simulink model "GCI_Ctrl_PLL_C2000"  (R2024a)
settings: Solver=FixedStepDiscrete  StartTime=0.0  StopTime=8  FixedStep=Sim.ContSampleTime  RelTol=1e-3  EnableMultiTasking=on
values from neighbouring files (symbols this model uses):
  ADPTV = 1.3912    [ModelDD.sldd]
  Ctrl = 0    [ModelDD.sldd]
  EnableMonitors = 0    [ModelDD.sldd]
  FrcPwr = 1    [ModelDD.sldd]
  IdSp = 0.0    [ModelDD.sldd]
  IqSp = 0.0    [ModelDD.sldd]
  ModReq = 1    [ModelDD.sldd]
  PorISel = 0    [ModelDD.sldd]
  PSp = 0.0    [ModelDD.sldd]
  QSp = 0.0    [ModelDD.sldd]
  Sim : value not decoded    [ModelDD.sldd]
  Test = 0    [ModelDD.sldd]
  Var = 650.0    [ModelDD.sldd]
undefined symbols (not defined in the file or in its folder): DiscIntNeverNeededParam, Down, GPTRIP1SEL, GPTRIP2SEL, magnitude, P, TZ1, TZ2, Up
libraries: simulink x38, c2837xDlib x22, c2802xlib x15, slpidlib x9, spsMeanLib x9, spsCurrentMeasurementLib x7, spsThreePhaseVIMeasurementLib x5, spsVoltageMeasurementLib x5, spsTHDLib x4, spsSeriesRLCBranchLib x4, svdutilitieslib x3, c280xlib x3
(part 2 of 11)

== system GCI_Ctrl_PLL_C2000/PowerSystem/Plant ==
  DutyIn : Inport
  Current Measurement : spsCurrentMeasurementLib/Current Measurement  PhasorSimulation=off  OutputType=Complex  PSBequivalent=0
  Current Measurement1 : spsCurrentMeasurementLib/Current Measurement  PhasorSimulation=off  OutputType=Complex  PSBequivalent=0
  Current Measurement2 : spsCurrentMeasurementLib/Current Measurement  PhasorSimulation=off  OutputType=Complex  PSBequivalent=0
  DC Voltage Source : spsDCVoltageSourceLib/DC Voltage Source  Amplitude=double(Var.HVDC.V)  Measurements=Voltage
  Data Type Conversion : DataTypeConversion  SaturateOnIntegerOverflow=off  RndMeth=Floor
  Data Type Conversion1 : DataTypeConversion  SaturateOnIntegerOverflow=off  RndMeth=Floor
  Ground : Ground
  Ground1 : spsGroundLib/Ground  LConnTagsString=a
  Measurment : Subsystem
  PWMGen1 : Subsystem  Commented=on  VariantControl=Var.Sim.SimOrHw == 1
  PWMGen2 : Subsystem  VariantControl=Var.Sim.SimOrHw == 1
  Series RLC Branch : spsSeriesRLCBranchLib/Series RLC Branch  LConnTagsString=__new0  RConnTagsString=__new0  BranchType=RC  Resistance=double(Var.HVDC.Cesr)  Inductance=1e-3  SetiL0=off  InitialCurrent=0  Capacitance=double(Var.HVDC.C)  Setx0=off  InitialVoltage=0  Measurements=Branch voltage and current
  Series RLC Branch1 : spsSeriesRLCBranchLib/Series RLC Branch  LConnTagsString=__new0  RConnTagsString=__new0  BranchType=RL  Resistance=double(Var.HVDC.Lesr)  Inductance=double(Var.HVDC.L)  SetiL0=off  InitialCurrent=0  Capacitance=Var.HVDC.C  Setx0=off  InitialVoltage=0  Measurements=Branch voltage and current
  Three-Phase Programmable Voltage Source1 : spsThreePhaseProgrammableVoltageSourceLib/Three-Phase Programmable Voltage Source  PositiveSequence="[double(Var.Grid.VphRms)*sqrt(3)  0 double(Var.Grid.Frq)]"  VariationEntity=Amplitude  VariationType=Table of time-amplitude pairs  VariationTypeAlt=Step  VariationStep=-20  VariationRate=10  VariationMagnitude=0.3  VariationFrequency=2  VariationTiming=[1 2]  VariationPhaseA=on  Amplitudes=[1 0.2 1]  TimeValues=[0 0.1 100]  HarmonicGeneration=on  HarmonicA=[3 0.05 -25 0]  HarmonicB=[5 0.05 35 0]  Timing="[0  110]"  BusType=swing  Pref=0  Qref=0  Qmin=-inf  Qmax=inf
  Three-Phase Series RLC Branch : spsThreePhaseSeriesRLCBranchLib/Three-Phase Series RLC Branch  LConnTagsString=A|B|C  RConnTagsString=A|B|C  BranchType=RL  Resistance=double(Var.Inductor.R)  Inductance=double(Var.Inductor.L)  Capacitance=1e-6  Measurements=Branch voltages and currents
  Three-Phase V-I Measurement1 : spsThreePhaseVIMeasurementLib/Three-Phase V-I Measurement  VoltageMeasurement=phase-to-ground  SetLabelV=on  LabelV=Vgrid_Ls  Vpu=off  VpuLL=off  CurrentMeasurement=no  SetLabelI=off  LabelI=Igrid_Ls  Ipu=off  Pbase=100e6  Vbase=500e3  OutputType=Complex  PhasorSimulation=off  PSBequivalent=0
  Three-Phase V-I Measurement4 : spsThreePhaseVIMeasurementLib/Three-Phase V-I Measurement  VoltageMeasurement=phase-to-ground  SetLabelV=on  LabelV=Vinv  Vpu=off  VpuLL=off  CurrentMeasurement=yes  SetLabelI=on  LabelI=Iinv  Ipu=off  Pbase=100e6  Vbase=500e3  OutputType=Complex  PhasorSimulation=off  PSBequivalent=0
  Two-Level Converter : spsTwoLevelConverterLib/Two-Level Converter  ModelType=Switching devices  Ron=1e-3  Rs=1e6  Cs=inf  Vforward=[0,0]  Ron_Diode=1e-3  Rs_Diode=1e6  Cs_Diode=inf  Vf_Diode=1e-3  Rs_CurrentSource=inf  Ron_ACsource=1e-3
      settings: LibrarySourceBlock=sps_lib/Power Electronics/Two-Level Converter
  Voltage Measurement : spsVoltageMeasurementLib/Voltage Measurement  PhasorSimulation=off  OutputType=Complex  PSBequivalent=0
  Voltage Measurement1 : spsVoltageMeasurementLib/Voltage Measurement  PhasorSimulation=off  OutputType=Complex  PSBequivalent=0
  powergui1 : spspowerguiLib/powergui  Priority=1  SimulationMode=Discrete  SampleTime=Sim.ContSampleTime  frequency=60  Iterations=50  frequencyindice=0  Pbase=100e6  ErrMax=1e-4  UnitsV=kV  UnitsW=MW  buscounter=0  FunctionMessages=off  echomessages=off  EnableUseOfTLC=off  CurrentSourceSwitches=off  DisableSnubberDevices=off  DisableRonSwitches=off  DisableVfSwitches=off  DisplayEquations=off  AutomaticDiscreteSolvers=off  SolverType=Tustin/Backward Euler (TBE)  Interpol=off  ExternalGateDelay=off  methode=off  Ts=100  x0status=blocks  SPID=off  SwTol=0  HookPort=off  NonlinearTolerance=1e-4  nMaxIteration=100  ContinueOnMaxIteration=off  RestoreLinks=warning  ResistiveCurrentMeasurement=off  Frange=[0:2:500]  Ylog=off  Xlog=on  ShowGrid=off  save=off  variable=ZData  structure=ScopeData2  ZoomFFT=off  StartTime=4.2  cycles=50  DisplayStyle=3  fundamental=46.5  FreqAxis=on  MaxFrequency=inf  frequencyindicesteady=1  RmsSteady=1  display=off
  MCU : Outport  VectorParamsAs1DForOutWhenUnconnected=off
  wires:
  [Vbat] -> Measurment/7(Vbat)
  [IhvdcCap] -> Measurment/6(Ihvdc_capa)
  Voltage Measurement/1 -> [Vbat]
  Data Type Conversion/1 -> MCU/1
  Current Measurement1/1 -> [IhvdcCap]
  [Ibat] -> Measurment/8(Ibat)
  [Vinv] -> Measurment/4(Vinv_abc)  "Vinv_abc"
  Measurment/1(MCU) -> Data Type Conversion/1
  [Ihvdc] -> Measurment/3(I_HVDC)  "I_HVD"
  [Vhvdc] -> Measurment/2(V_HVDC)  "V_HVD"
  [Vgrid_Ls] -> Measurment/1(Vgrid_abc)  "Vgrid_abc"
  DutyIn/1 -> PWMGen2/1(Duty)
  Data Type Conversion1/1 -> Two-Level Converter/1
  Ground/1 -> Two-Level Converter/2
  Current Measurement/1 -> [Ihvdc]
  Voltage Measurement1/1 -> [Vhvdc]
  [Iinv] -> Measurment/5(Iinv_abc)  "Iinv_abc"
  Current Measurement2/1 -> [Ibat]
  PWMGen2/1(PWM) -> Data Type Conversion1/1
  connections:
  Three-Phase V-I Measurement4/RConn1 -- Three-Phase Series RLC Branch/LConn1
  Three-Phase V-I Measurement1/RConn1 -- Three-Phase Series RLC Branch/RConn1
  DC Voltage Source/LConn1 -- Voltage Measurement1/LConn2 -- Voltage Measurement/LConn2 -- Series RLC Branch/RConn1 -- Two-Level Converter/RConn2
  Current Measurement/RConn1 -- Two-Level Converter/RConn1
  Three-Phase V-I Measurement4/LConn3 -- Two-Level Converter/LConn3
  Three-Phase V-I Measurement4/RConn2 -- Three-Phase Series RLC Branch/LConn2
  Three-Phase V-I Measurement1/RConn3 -- Three-Phase Series RLC Branch/RConn3
  Three-Phase V-I Measurement1/RConn2 -- Three-Phase Series RLC Branch/RConn2
  Current Measurement2/LConn1 -- Series RLC Branch1/RConn1
  DC Voltage Source/RConn1 -- Series RLC Branch1/LConn1 -- Voltage Measurement/LConn1
  Current Measurement/LConn1 -- Voltage Measurement1/LConn1 -- Current Measurement2/RConn1 -- Current Measurement1/LConn1
  Three-Phase V-I Measurement4/LConn1 -- Two-Level Converter/LConn1
  Three-Phase V-I Measurement4/LConn2 -- Two-Level Converter/LConn2
  Current Measurement1/RConn1 -- Series RLC Branch/LConn1
  Three-Phase V-I Measurement4/RConn3 -- Three-Phase Series RLC Branch/LConn3
  Three-Phase Programmable Voltage Source1/RConn3 -- Three-Phase V-I Measurement1/LConn3
  Three-Phase Programmable Voltage Source1/RConn2 -- Three-Phase V-I Measurement1/LConn2
  Three-Phase Programmable Voltage Source1/LConn1 -- Ground1/LConn1
  Three-Phase V-I Measurement1/LConn1 -- Three-Phase Programmable Voltage Source1/RConn1

== system GCI_Ctrl_PLL_C2000/C2000_SW/Control/CommunicationMode ==
  HWI_SCIA_RX_INT : svdschedulerlib/Hardware Interrupt v2  ISRGroup=ADC - Analog to Digital Converter  ISRName=ADCA1_INT  ISRNumber=32  NumEventsToServe=1  EventsList=[{'on','EOC event','1'};{'off','Overflow event','2'};{'off','Custom event','3'};{'off','Default event','4'}]  SelectedEvents={'event1'}  TaskPriority=50  DisablePreemption=on  ClearInterruptFlagsAtEndOfEvent=on  InterruptDefinitionFile=$(TARGET_ROOT)/registry/interrupts/F2837xS_interrupts.xml  HardwareBoard=F2837x  EnableSimPort=off
      settings: LibrarySourceBlock=c2000lib/Scheduling/Hardware Interrupt
  Serial Receive : Subsystem  SystemSampleTime=1e-3
  wires:
  HWI_SCIA_RX_INT/1 -> Serial Receive/Trigger

== system GCI_Ctrl_PLL_C2000/C2000_SW/Control/ExternalMode ==
  Constant : Constant  Commented=on  Value=Ctrl.IdSp  OutDataTypeStr=single  SampleTime=10/double(Var.PWM_Freq)
  Constant1 : Constant  Commented=on  Value=Ctrl.IqSp  OutDataTypeStr=single  SampleTime=10/double(Var.PWM_Freq)
  Constant10 : Constant  Value=IdSp  OutDataTypeStr=single  SampleTime=10/double(Var.PWM_Freq)
  Constant11 : Constant  Value=IqSp  OutDataTypeStr=single  SampleTime=10/double(Var.PWM_Freq)
  Constant12 : Constant  Value=PorISel  SampleTime=10/double(Var.PWM_Freq)
  Constant13 : Constant  Value=PSp  OutDataTypeStr=single  SampleTime=10/double(Var.PWM_Freq)
  Constant14 : Constant  Value=Ctrl.EnPll  SampleTime=10/double(Var.PWM_Freq)
  Constant15 : Constant  Value=QSp  OutDataTypeStr=single  SampleTime=10/double(Var.PWM_Freq)
  Constant16 : Constant  Value=EnableMonitors  SampleTime=10/double(Var.PWM_Freq)
  Constant17 : Constant  Value=Test  SampleTime=10/double(Var.PWM_Freq)
  Constant18 : Constant  Value=FrcPwr  SampleTime=10/double(Var.PWM_Freq)
  Constant19 : Constant  Value=ModReq  SampleTime=10/double(Var.PWM_Freq)
  Constant2 : Constant  Commented=on  Value=Ctrl.PorISel  OutDataTypeStr=boolean  SampleTime=10/double(Var.PWM_Freq)
  Constant3 : Constant  Commented=on  Value=Ctrl.PSp  OutDataTypeStr=single  SampleTime=10/double(Var.PWM_Freq)
  Constant4 : Constant  Commented=on  Value=Ctrl.EnPll  OutDataTypeStr=boolean  SampleTime=10/double(Var.PWM_Freq)
  Constant5 : Constant  Commented=on  Value=Ctrl.QSp  OutDataTypeStr=single  SampleTime=10/double(Var.PWM_Freq)
  Constant6 : Constant  Commented=on  Value=Ctrl.EnableMonitors  OutDataTypeStr=boolean  SampleTime=10/double(Var.PWM_Freq)
  Constant7 : Constant  Commented=on  Value=Ctrl.Test  OutDataTypeStr=boolean  SampleTime=10/double(Var.PWM_Freq)
  Constant8 : Constant  Commented=on  Value=Ctrl.FrcPwr  OutDataTypeStr=boolean  SampleTime=10/double(Var.PWM_Freq)
  Constant9 : Constant  Commented=on  Value=Ctrl.ModReq  OutDataTypeStr=boolean  SampleTime=10/double(Var.PWM_Freq)
  Data Store Write : DataStoreWrite  Commented=on  DataStoreName=FrcPwr  IndexOptions=Index vector (dialog)  Indices=1  OutputSizes=1
  Data Store Write1 : DataStoreWrite  Commented=on  DataStoreName=TestTrig  IndexOptions=Index vector (dialog)  Indices=1  OutputSizes=1
  Data Store Write10 : DataStoreWrite  DataStoreName=FrcPwr  IndexOptions=Index vector (dialog)  Indices=1  OutputSizes=1
  Data Store Write11 : DataStoreWrite  DataStoreName=TestTrig  IndexOptions=Index vector (dialog)  Indices=1  OutputSizes=1
  Data Store Write12 : DataStoreWrite  DataStoreName=ModReq  IndexOptions=Index vector (dialog)  Indices=1  OutputSizes=1
  Data Store Write13 : DataStoreWrite  DataStoreName=EnaMon  IndexOptions=Index vector (dialog)  Indices=1  OutputSizes=1
  Data Store Write14 : DataStoreWrite  DataStoreName=EnaPLL  IndexOptions=Index vector (dialog)  Indices=1  OutputSizes=1
  Data Store Write15 : DataStoreWrite  DataStoreName=Sel_P_I  IndexOptions=Index vector (dialog)  Indices=1  OutputSizes=1
  Data Store Write16 : DataStoreWrite  DataStoreName=IdSp  IndexOptions=Index vector (dialog)  Indices=1  OutputSizes=1
  Data Store Write17 : DataStoreWrite  DataStoreName=IqSp  IndexOptions=Index vector (dialog)  Indices=1  OutputSizes=1
  Data Store Write18 : DataStoreWrite  DataStoreName=PSp  IndexOptions=Index vector (dialog)  Indices=1  OutputSizes=1
  Data Store Write19 : DataStoreWrite  DataStoreName=QSp  IndexOptions=Index vector (dialog)  Indices=1  OutputSizes=1
  Data Store Write2 : DataStoreWrite  Commented=on  DataStoreName=ModReq  IndexOptions=Index vector (dialog)  Indices=1  OutputSizes=1
  Data Store Write3 : DataStoreWrite  Commented=on  DataStoreName=EnaMon  IndexOptions=Index vector (dialog)  Indices=1  OutputSizes=1
  Data Store Write4 : DataStoreWrite  Commented=on  DataStoreName=EnaPLL  IndexOptions=Index vector (dialog)  Indices=1  OutputSizes=1
  Data Store Write5 : DataStoreWrite  Commented=on  DataStoreName=Sel_P_I  IndexOptions=Index vector (dialog)  Indices=1  OutputSizes=1
  Data Store Write6 : DataStoreWrite  Commented=on  DataStoreName=IdSp  IndexOptions=Index vector (dialog)  Indices=1  OutputSizes=1
  Data Store Write7 : DataStoreWrite  Commented=on  DataStoreName=IqSp  IndexOptions=Index vector (dialog)  Indices=1  OutputSizes=1
  Data Store Write8 : DataStoreWrite  Commented=on  DataStoreName=PSp  IndexOptions=Index vector (dialog)  Indices=1  OutputSizes=1
  Data Store Write9 : DataStoreWrite  Commented=on  DataStoreName=QSp  IndexOptions=Index vector (dialog)  Indices=1  OutputSizes=1
  Manual Switch : ManualSwitch
  Manual Switch1 : ManualSwitch
  Manual Switch2 : ManualSwitch  CurrentSetting=0
  Signal Editor : SignalEditorBlockLib/Signal Editor  FileName=PQ_SP.mat  ActiveScenario=PQ2  ActiveSignal=P*  IsBus=off  OutputBusObjectStr=Bus: BusObject  SampleTime=10/double(Var.PWM_Freq)  ZeroCross=off  OutputAfterFinalValue=Setting to zero  Unit=inherit  PreserveSignalName=on  ApplySigPropsToAllScenarios=on  ApplySigPropsToAllSignals=on
  Step : Step  SampleTime=10/double(Var.PWM_Freq)
  wires:
  Constant/1 -> Data Store Write6/1
  Constant1/1 -> Data Store Write7/1
  Constant3/1 -> Data Store Write8/1
  Constant5/1 -> Data Store Write9/1
  Constant2/1 -> Data Store Write5/1
  Constant7/1 -> Data Store Write1/1
  Constant6/1 -> Data Store Write3/1
  Constant4/1 -> Data Store Write4/1
  Constant19/1 -> Data Store Write12/1
  Constant18/1 -> Data Store Write10/1
  Signal Editor/2 -> Manual Switch1/2
  Constant10/1 -> Data Store Write16/1
  Constant16/1 -> Data Store Write13/1
  Constant11/1 -> Data Store Write17/1
  Signal Editor/1 -> Manual Switch/2
  Constant12/1 -> Data Store Write15/1
  Constant17/1 -> Manual Switch2/1
  Constant14/1 -> Data Store Write14/1
  Constant8/1 -> Data Store Write/1
  Constant9/1 -> Data Store Write2/1
  Constant13/1 -> Manual Switch/1
  Manual Switch/1 -> Data Store Write18/1
  Constant15/1 -> Manual Switch1/1
  Manual Switch1/1 -> Data Store Write19/1
  Step/1 -> Manual Switch2/2
  Manual Switch2/1 -> Data Store Write11/1

== system GCI_Ctrl_PLL_C2000/C2000_SW/CtrlLoop/ADC Scaling ==
  Ch1 : Inport
  Ch2 : Inport  Port=2
  Ch3 : Inport  Port=3
  Ch4 : Inport  Port=4
  Ch5 : Inport  Port=5
  Ch6 : Inport  Port=6
  SPO : Inport  Port=7
  PllEn : Inport  Port=8
  ADC Scaling 3 Cur : Subsystem  Priority=2  VariantControl="Sim.ADC_UabcSensor == \"Three Currents\""
  ADC Scaling 3 Volts : Subsystem  Priority=2  VariantControl="Sim.ADC_UabcSensor == \"Three Volts\""
  Vgrid_abc : Outport  Unit=V  VectorParamsAs1DForOutWhenUnconnected=off
  I_abc : Outport  Port=2  Unit=A  VectorParamsAs1DForOutWhenUnconnected=off
  Vhvdc : Outport  Port=3  VectorParamsAs1DForOutWhenUnconnected=off
  Mon : Outport  Port=4  VectorParamsAs1DForOutWhenUnconnected=off

== system GCI_Ctrl_PLL_C2000/C2000_SW/CtrlLoop/ADCs ==
  Meas : Inport
  HW : Subsystem  Priority=2  VariantControl="Sim.SimOrHw == \"Hw\""
  SIM : Subsystem  Priority=2  VariantControl="Sim.SimOrHw == \"Sim\""
  A_Ch2 : Outport  VectorParamsAs1DForOutWhenUnconnected=off
  B_Ch2 : Outport  Port=2  VectorParamsAs1DForOutWhenUnconnected=off
  C_Ch2 : Outport  Port=3  VectorParamsAs1DForOutWhenUnconnected=off
  A_Ch3 : Outport  Port=4  VectorParamsAs1DForOutWhenUnconnected=off
  B_Ch3 : Outport  Port=5  VectorParamsAs1DForOutWhenUnconnected=off
  C_Ch3 : Outport  Port=6  VectorParamsAs1DForOutWhenUnconnected=off
  ADCs : Outport  Port=7  VectorParamsAs1DForOutWhenUnconnected=off

== system GCI_Ctrl_PLL_C2000/C2000_SW/CtrlLoop/CurrentController ==
  Enable : Inport
  Vdc : Inport  Port=2
  VabcGridAdj : Inport  Port=3
  VdqPll : Inport  Port=4
  wtNow : Inport  Port=5
  wtNext : Inport  Port=6
  w : Inport  Port=7
  Iabc : Inport  Port=8
  CurrentController : Subsystem  VariantControl=Sim.CC_Enable == 1
  CurrentControllerAdptv : Subsystem  VariantControl=Sim.CC_Enable== 3
  CurrentControllerAdptv2 : Subsystem  VariantControl=Sim.CC_Enable== 4
  CurrentControllerPosNegSeq : Subsystem  VariantControl=Sim.CC_Enable== 2
  FeedForward : Subsystem  VariantControl=Sim.CC_Enable== 0
  VabcRef : Outport  Unit=V  VectorParamsAs1DForOutWhenUnconnected=off
  Mon : Outport  Port=2  VectorParamsAs1DForOutWhenUnconnected=off

== system GCI_Ctrl_PLL_C2000/C2000_SW/CtrlLoop/LPF2 ==
  u : Inport
  Alpha : Gain  Gain=(2-w*Ts)/(2+w*Ts)
  Beta : Gain  Gain=(w*Ts)/(2+w*Ts)
  Delay1 : Delay  DelayLength=1  InitialCondition=y_0
  Delay2 : Delay  DelayLength=1
  Sum1 : Sum  Inputs=++|
  Sum2 : Sum  Inputs=|++
  y : Outport  VectorParamsAs1DForOutWhenUnconnected=off
  wires:
  Sum2/1 -> y/1, Delay1/1  "VdcActRms"
  Beta/1 -> Sum2/1
  Sum1/1 -> Beta/1
  Delay2/1 -> Sum1/2
  Alpha/1 -> Sum2/2
  Delay1/1 -> Alpha/1  "y(n-1)"
  u/1 -> Delay2/1, Sum1/1

== system GCI_Ctrl_PLL_C2000/C2000_SW/CtrlLoop/Modulation ==
  Enable : Inport
  Vdc : Inport  Port=2
  VabcSp : Inport  Port=3
  M_Adaptive : Subsystem  VariantControl="Sim.Modulation == \"Adaptive\""
  SPWM : Subsystem  Priority=2  VariantControl="Sim.Modulation == \"SPWM\""
  SVM : Subsystem  VariantControl="Sim.Modulation == \"SVPWM\""
  Duty : Outport  Unit=%  VectorParamsAs1DForOutWhenUnconnected=off
  Mon : Outport  Port=2  VectorParamsAs1DForOutWhenUnconnected=off

== system GCI_Ctrl_PLL_C2000/C2000_SW/CtrlLoop/Observer ==
  VabcInv : Inport
  VabcGrid : Inport  Port=2
  Enable : EnablePort
  Bus Selector : BusSelector  OutputSignals=VabcGrid,wtCur
  Bus Selector1 : BusSelector  OutputSignals=VabcAct
  Delay{1..2,5..7} (5 alike) : Delay  DelayLength=1
  Delay4 : Delay
  Discrete-Time Integrator1 : DiscreteIntegrator  IntegratorMethod=Integration: Trapezoidal  gainval=single(1)  ExternalReset=either  InitialCondition=single(0)  SampleTime=-1  LimitOutput=on  UpperSaturationLimit=1000  LowerSaturationLimit=-1000  ShowSaturationPort=on  ICPrevOutput=DiscIntNeverNeededParam  ICPrevScaledInput=DiscIntNeverNeededParam
  Discrete-Time Integrator2 : DiscreteIntegrator  IntegratorMethod=Integration: Trapezoidal  gainval=single(1)  ExternalReset=either  InitialCondition=single(0)  SampleTime=-1  LimitOutput=on  UpperSaturationLimit=1000  LowerSaturationLimit=-1000  ShowSaturationPort=on  ICPrevOutput=DiscIntNeverNeededParam  ICPrevScaledInput=DiscIntNeverNeededParam
  Gain : Gain  Gain=Var.Inductor_R +Var.Transformer.R1+Var.Transformer.R2
  Gain1 : Gain  Gain=1/Var.Transformer.Rc  ParamDataTypeStr=single
  Gain11 : Gain  ParamDataTypeStr=single
  Gain2 : Gain  Gain=1/Var.Transformer.Lm  ParamDataTypeStr=single
  Gain3 : Gain  Gain=1/(Var.Inductor_L+Var.Transformer.L1+Var.Transformer.L2)  ParamDataTypeStr=single
  Gain4 : Gain  Gain=1/Var.Transformer.N  ParamDataTypeStr=single
  Gain5 : Gain  Commented=on  Gain=1/Var.Transformer.N  ParamDataTypeStr=single
  LPF : Subsystem  VariantControl=Var.Pll.FiltDcOff == 1
  LPF1 : Subsystem  VariantControl=Var.Pll.FiltDcOff == 1
  Scope : Scope  NumInputPorts=3
  Sum : Sum  Inputs=-+|
  Sum of Elements : Sum  Inputs=+
  Sum of Elements1 : Sum  Inputs=+
  Sum1 : Sum  Inputs=|+-
  Sum2 : Sum  Inputs=--+||
  Terminator : Terminator
  wires:
  Sum of Elements1/1 -> Discrete-Time Integrator1/2
  Gain1/1 -> Sum2/1
  Delay1/1 -> Gain/1
  Gain3/1 -> Discrete-Time Integrator2/1
  Delay5/1 -> Gain11/1
  Discrete-Time Integrator1/2 -> Delay2/1
  Gain11/1 -> Gain1/1, Sum/1, Gain2/1
  Discrete-Time Integrator2/1 -> Sum2/3, LPF1/1(VabcGrid)
  Sum/1 -> Sum1/1
  Sum2/1 -> Gain4/1
  Delay4/1 -> Sum/2
  Discrete-Time Integrator1/1 -> Sum2/2
  Gain/1 -> Sum1/2
  Sum1/1 -> Gain3/1
  Discrete-Time Integrator2/2 -> Delay7/1
  Delay2/1 -> Sum of Elements1/1
  Gain2/1 -> Discrete-Time Integrator1/1
  Sum of Elements/1 -> Discrete-Time Integrator2/2
  VabcGrid/1 -> Bus Selector/1
  Delay7/1 -> Sum of Elements/1
  Bus Selector/1 -> Delay5/1  "<VabcGrid>"
  VabcInv/1 -> Bus Selector1/1
  Bus Selector1/1 -> Delay4/1  "<VabcAct>"
  Gain4/1 -> Scope/1, LPF/1(VabcGrid)
  Bus Selector/2 -> Delay6/1  "<wtCur>"
  Delay6/1 -> [wt]
  LPF/1(VabcGridAdj) -> Scope/2, Terminator/1
  LPF1/1(VabcGridAdj) -> Delay1/1, Scope/3

== system GCI_Ctrl_PLL_C2000/C2000_SW/CtrlLoop/PLL_Vref ==
  note: Data Collection
  VabcGrid : Inport
  Iabc : Inport  Port=2
  Enable : EnablePort  StatesWhenEnabling=reset
  Bus Creator : BusCreator  Inputs=11
  Delay2 : Delay  DelayLength=1
  Gain : Gain
  Gain1 : Gain  Commented=on  Gain=(1/sqrt(3))*1/Var.Transformer_N
  Manual Switch : ManualSwitch  CurrentSetting=0
  SRF_PLL : Subsystem
  Subsystem : Subsystem
  abc2dqzFilt : Subsystem  Variant=on  VariantControl=Variant1
  VdqzGridAdj : Outport  Unit=V  VectorParamsAs1DForOutWhenUnconnected=off
  VdqPll : Outport  Port=2  Unit=V  VectorParamsAs1DForOutWhenUnconnected=off
  wtNow : Outport  Port=3  Unit=rad  VectorParamsAs1DForOutWhenUnconnected=off
  wtNext : Outport  Port=4  Unit=rad  VectorParamsAs1DForOutWhenUnconnected=off
  w : Outport  Port=5  Unit=rad/s  VectorParamsAs1DForOutWhenUnconnected=off
  Synch : Outport  Port=6  VectorParamsAs1DForOutWhenUnconnected=off
  Mon : Outport  Port=7  VectorParamsAs1DForOutWhenUnconnected=off
  wires:
  abc2dqzFilt/2(dqz_Pll) -> [VdqzPll], SRF_PLL/1(Vdqz)  "Vdqz_Pll"
  [wtNext] -> Delay2/1
  Delay2/1 -> abc2dqzFilt/2(Ang)  "wtCur"
  SRF_PLL/4(wFilt) -> [wFilt]
  SRF_PLL/1(wtNext) -> [wtNext]
  [Vdqz] -> Bus Creator/3
  [wtNext] -> Bus Creator/7
  [wtCur] -> Bus Creator/8  "wtCur"
  Bus Creator/1 -> Mon/1  "PllMon"
  [w] -> Bus Creator/9
  [VabcGrid] -> Bus Creator/1  "VabcGrid"
  SRF_PLL/3(w) -> [w]
  [wFilt] -> Bus Creator/10
  [VabcGridAdj] -> Bus Creator/2  "VabcGridAdj"
  [w] -> Manual Switch/2
  abc2dqzFilt/1(Dqz) -> [Vdqz]  "Vdqz"
  [VdqzPll] -> Bus Creator/4
  [w] -> w/1
  [VabcGridAdj] -> VdqzGridAdj/1
  SRF_PLL/2(wtNow) -> [wtCur]
  [wtNext] -> wtNext/1
  [wtCur] -> wtNow/1
  Manual Switch/1 -> abc2dqzFilt/3(w)
  SRF_PLL/5(Snch) -> [Synch]
  [Synch] -> Synch/1
  [wFilt] -> Manual Switch/1
  [wtCur] -> Subsystem/3(wtNow)
  [Iabc] -> Subsystem/2(Iabc)
  Iabc/1 -> [Iabc]
  Subsystem/1(PQ) -> [PQ]  "PQ"
  Subsystem/2(Idqz) -> [Idqz]  "Idqz"
  [Idqz] -> Bus Creator/5  "Idqz"
  [PQ] -> Bus Creator/6
  [Synch] -> Bus Creator/11
  [VdqzPll] -> VdqPll/1
  VabcGrid/1 -> Gain/1, [VabcGrid]
  Gain/1 -> [VabcGridAdj], abc2dqzFilt/1(abc)
  [VabcGridAdj] -> Subsystem/1(Vabc)

== system GCI_Ctrl_PLL_C2000/C2000_SW/CtrlLoop/PWMs ==
  Duty : Inport
  SPO : Inport  Port=2
  HW : Subsystem  Priority=2  VariantControl="Sim.SimOrHw ==  \"Hw\""
  SIM : Subsystem  Priority=2  VariantControl="Sim.SimOrHw == \"Sim\""
  DutyOut : Outport  VectorParamsAs1DForOutWhenUnconnected=off

== system GCI_Ctrl_PLL_C2000/C2000_SW/CtrlLoop/RMS ==
  abc : Inport
  LPF2 : Subsystem  mask{Ts=1/(Var.PWM_Freq), w=single(2*pi*10), K=single(1), y_0=single(2*pi*Var.Grid_Frq)}
      mask prompts: Ts "Sample Time (s)"; w "CutOff Freq (-3db) (rad/s)"; K "Gain"; y_0 "Initial output"
  Sqrt1 : Sqrt
  Square : Math  Operator=square
  CalcRms : Outport
  wires:
  LPF2/1(y) -> Sqrt1/1
  abc/1 -> Square/1
  Square/1 -> LPF2/1(u)
  Sqrt1/1 -> CalcRms/1  "IabcActRms"

== system GCI_Ctrl_PLL_C2000/C2000_SW/CtrlLoop/RMS1 ==
  abc : Inport
  LPF2 : Subsystem  mask{Ts=1/(Var.PWM_Freq), w=single(2*pi*1), K=single(1), y_0=single(2*pi*Var.Grid_Frq)}
      mask prompts: Ts "Sample Time (s)"; w "CutOff Freq (-3db) (rad/s)"; K "Gain"; y_0 "Initial output"
  Sqrt1 : Sqrt
  Square : Math  Operator=square
  CalcRms : Outport
  wires:
  Sqrt1/1 -> CalcRms/1  "VgabcActRms"
  Square/1 -> LPF2/1(u)
  abc/1 -> Square/1
  LPF2/1(y) -> Sqrt1/1

== system GCI_Ctrl_PLL_C2000/C2000_SW/ISR_CtrlLoop/HW ==
  C28x Hardware Interrupt : c2000lib/Scheduling/C28x Hardware Interrupt  irqnumbers=[3]  pienumbers=[4]  irqpriorities=[1]  irqpreempts=[1]  showinput=off  dspchiptype=C280X
  Intrupt : Outport  VectorParamsAs1DForOutWhenUnconnected=off
  wires:
  C28x Hardware Interrupt/1 -> Intrupt/1  "CtrlInt"

== system GCI_Ctrl_PLL_C2000/C2000_SW/ISR_CtrlLoop/SIM ==
  Function-Call Generator : simulink/Ports & Subsystems/Function-Call Generator  sample_time=1/double(Var.PWM_Freq)  numberOfIterations=1  DisallowWideOutput=off
  Intrupt : Outport  VectorParamsAs1DForOutWhenUnconnected=off
  wires:
  Function-Call Generator/1 -> Intrupt/1  "CtrlInt"

== system GCI_Ctrl_PLL_C2000/C2000_SW/ISR_MnrErr/HW ==
  C28x Hardware Interrupt : c2000lib/Scheduling/C28x Hardware Interrupt  Commented=on  irqnumbers=[3]  pienumbers=[4]  irqpriorities=[1]  irqpreempts=[1]  showinput=off  dspchiptype=C280X
  Function-Call Generator : simulink/Ports & Subsystems/Function-Call Generator  sample_time=10/double(Var.PWM_Freq)  numberOfIterations=1  DisallowWideOutput=off
  Intrupt : Outport  VectorParamsAs1DForOutWhenUnconnected=off
  wires:
  Function-Call Generator/1 -> Intrupt/1  "MonInt"

== system GCI_Ctrl_PLL_C2000/C2000_SW/ISR_MnrErr/SIM ==
  Function-Call Generator : simulink/Ports & Subsystems/Function-Call Generator  sample_time=2/double(Var.PWM_Freq)  numberOfIterations=1  DisallowWideOutput=off
  Intrupt : Outport  VectorParamsAs1DForOutWhenUnconnected=off
  wires:
  Function-Call Generator/1 -> Intrupt/1  "MonInt"

== system GCI_Ctrl_PLL_C2000/C2000_SW/ISR_SysSts/HW ==
  C28x Hardware Interrupt : c2000lib/Scheduling/C28x Hardware Interrupt  Commented=on  irqnumbers=[3]  pienumbers=[4]  irqpriorities=[1]  irqpreempts=[1]  showinput=off  dspchiptype=C280X
  Function-Call Generator : simulink/Ports & Subsystems/Function-Call Generator  sample_time=10/double(Var.PWM_Freq)  numberOfIterations=1  DisallowWideOutput=off
  Intrupt : Outport  VectorParamsAs1DForOutWhenUnconnected=off
  wires:
  Function-Call Generator/1 -> Intrupt/1  "SysStsInt"

== system GCI_Ctrl_PLL_C2000/C2000_SW/ISR_SysSts/SIM ==
  Function-Call Generator : simulink/Ports & Subsystems/Function-Call Generator  sample_time=10/double(Var.PWM_Freq)  numberOfIterations=1  DisallowWideOutput=off
  Intrupt : Outport  VectorParamsAs1DForOutWhenUnconnected=off
  wires:
  Function-Call Generator/1 -> Intrupt/1  "SysStsInt"

== system GCI_Ctrl_PLL_C2000/C2000_SW/MnrErr/HwFaults ==
  note: Over-Temprature Protection
  note: Short Circuit Protection
  note: Over-Voltage Protection
  note: Over-Current Protection
  note: GPIO 22
  note: GPIO 104
  note: GPIO 105
  note: GPIO 124
  note: GPIO 125
  note: GPIO 95
  note: GPIO 32
  note: GPIO 56
  Data Type Conversion{,1..5} (6 alike) : DataTypeConversion  OutDataTypeStr=boolean  SaturateOnIntegerOverflow=off  RndMeth=Floor
  Digital Input : c2837xDlib/Digital Input  GPIO_Number=GPIO32~GPIO39  GPIO_Bit0=on  GPIO_Bit1=off  GPIO_Bit2=off  GPIO_Bit3=off  GPIO_Bit4=off  GPIO_Bit5=off  GPIO_Bit6=off  GPIO_Bit7=off  sampleTime=-1  dataType=auto  GPIO_Bit0_Qualification=Sync to SYSCLKOUT  GPIO_Bit1_Qualification=Sync to SYSCLKOUT  GPIO_Bit2_Qualification=Sync to SYSCLKOUT  GPIO_Bit3_Qualification=Sync to SYSCLKOUT  GPIO_Bit4_Qualification=Sync to SYSCLKOUT  GPIO_Bit5_Qualification=Sync to SYSCLKOUT  GPIO_Bit6_Qualification=Sync to SYSCLKOUT  GPIO_Bit7_Qualification=Sync to SYSCLKOUT  Qualification_Period=-1
  Digital Input1 : c2837xDlib/Digital Input  GPIO_Number=GPIO16~GPIO23  GPIO_Bit0=off  GPIO_Bit1=off  GPIO_Bit2=off  GPIO_Bit3=off  GPIO_Bit4=off  GPIO_Bit5=off  GPIO_Bit6=on  GPIO_Bit7=off  sampleTime=-1  dataType=auto  GPIO_Bit0_Qualification=Sync to SYSCLKOUT  GPIO_Bit1_Qualification=Sync to SYSCLKOUT  GPIO_Bit2_Qualification=Sync to SYSCLKOUT  GPIO_Bit3_Qualification=Sync to SYSCLKOUT  GPIO_Bit4_Qualification=Sync to SYSCLKOUT  GPIO_Bit5_Qualification=Sync to SYSCLKOUT  GPIO_Bit6_Qualification=Sync to SYSCLKOUT  GPIO_Bit7_Qualification=Sync to SYSCLKOUT  Qualification_Period=-1
  Digital Input2 : c2837xDlib/Digital Input  GPIO_Number=GPIO104~GPIO111  GPIO_Bit0=on  GPIO_Bit1=off  GPIO_Bit2=off  GPIO_Bit3=off  GPIO_Bit4=off  GPIO_Bit5=off  GPIO_Bit6=off  GPIO_Bit7=off  sampleTime=-1  dataType=auto  GPIO_Bit0_Qualification=Sync to SYSCLKOUT  GPIO_Bit1_Qualification=Sync to SYSCLKOUT  GPIO_Bit2_Qualification=Sync to SYSCLKOUT  GPIO_Bit3_Qualification=Sync to SYSCLKOUT  GPIO_Bit4_Qualification=Sync to SYSCLKOUT  GPIO_Bit5_Qualification=Sync to SYSCLKOUT  GPIO_Bit6_Qualification=Sync to SYSCLKOUT  GPIO_Bit7_Qualification=Sync to SYSCLKOUT  Qualification_Period=-1
  Digital Input3 : c2837xDlib/Digital Input  GPIO_Number=GPIO104~GPIO111  GPIO_Bit0=off  GPIO_Bit1=on  GPIO_Bit2=off  GPIO_Bit3=off  GPIO_Bit4=off  GPIO_Bit5=off  GPIO_Bit6=off  GPIO_Bit7=off  sampleTime=-1  dataType=auto  GPIO_Bit0_Qualification=Sync to SYSCLKOUT  GPIO_Bit1_Qualification=Sync to SYSCLKOUT  GPIO_Bit2_Qualification=Sync to SYSCLKOUT  GPIO_Bit3_Qualification=Sync to SYSCLKOUT  GPIO_Bit4_Qualification=Sync to SYSCLKOUT  GPIO_Bit5_Qualification=Sync to SYSCLKOUT  GPIO_Bit6_Qualification=Sync to SYSCLKOUT  GPIO_Bit7_Qualification=Sync to SYSCLKOUT  Qualification_Period=-1
  Digital Input4 : c2837xDlib/Digital Input  GPIO_Number=GPIO120~GPIO127  GPIO_Bit0=off  GPIO_Bit1=off  GPIO_Bit2=off  GPIO_Bit3=off  GPIO_Bit4=on  GPIO_Bit5=off  GPIO_Bit6=off  GPIO_Bit7=off  sampleTime=-1  dataType=auto  GPIO_Bit0_Qualification=Sync to SYSCLKOUT  GPIO_Bit1_Qualification=Sync to SYSCLKOUT  GPIO_Bit2_Qualification=Sync to SYSCLKOUT  GPIO_Bit3_Qualification=Sync to SYSCLKOUT  GPIO_Bit4_Qualification=Sync to SYSCLKOUT  GPIO_Bit5_Qualification=Sync to SYSCLKOUT  GPIO_Bit6_Qualification=Sync to SYSCLKOUT  GPIO_Bit7_Qualification=Sync to SYSCLKOUT  Qualification_Period=-1
  Digital Input5 : c2837xDlib/Digital Input  GPIO_Number=GPIO120~GPIO127  GPIO_Bit0=off  GPIO_Bit1=off  GPIO_Bit2=off  GPIO_Bit3=off  GPIO_Bit4=off  GPIO_Bit5=on  GPIO_Bit6=off  GPIO_Bit7=off  sampleTime=-1  dataType=auto  GPIO_Bit0_Qualification=Sync to SYSCLKOUT  GPIO_Bit1_Qualification=Sync to SYSCLKOUT  GPIO_Bit2_Qualification=Sync to SYSCLKOUT  GPIO_Bit3_Qualification=Sync to SYSCLKOUT  GPIO_Bit4_Qualification=Sync to SYSCLKOUT  GPIO_Bit5_Qualification=Sync to SYSCLKOUT  GPIO_Bit6_Qualification=Sync to SYSCLKOUT  GPIO_Bit7_Qualification=Sync to SYSCLKOUT  Qualification_Period=-1
  Digital Input6 : c2837xDlib/Digital Input  GPIO_Number=GPIO88~GPIO95  GPIO_Bit0=off  GPIO_Bit1=off  GPIO_Bit2=off  GPIO_Bit3=off  GPIO_Bit4=off  GPIO_Bit5=off  GPIO_Bit6=off  GPIO_Bit7=on  sampleTime=-1  dataType=auto  GPIO_Bit0_Qualification=Sync to SYSCLKOUT  GPIO_Bit1_Qualification=Sync to SYSCLKOUT  GPIO_Bit2_Qualification=Sync to SYSCLKOUT  GPIO_Bit3_Qualification=Sync to SYSCLKOUT  GPIO_Bit4_Qualification=Sync to SYSCLKOUT  GPIO_Bit5_Qualification=Sync to SYSCLKOUT  GPIO_Bit6_Qualification=Sync to SYSCLKOUT  GPIO_Bit7_Qualification=Sync to SYSCLKOUT  Qualification_Period=-1
  Digital Input7 : c2837xDlib/Digital Input  GPIO_Number=GPIO56~GPIO63  GPIO_Bit0=on  GPIO_Bit1=off  GPIO_Bit2=off  GPIO_Bit3=off  GPIO_Bit4=off  GPIO_Bit5=off  GPIO_Bit6=off  GPIO_Bit7=off  sampleTime=-1  dataType=auto  GPIO_Bit0_Qualification=Sync to SYSCLKOUT  GPIO_Bit1_Qualification=Sync to SYSCLKOUT  GPIO_Bit2_Qualification=Sync to SYSCLKOUT  GPIO_Bit3_Qualification=Sync to SYSCLKOUT  GPIO_Bit4_Qualification=Sync to SYSCLKOUT  GPIO_Bit5_Qualification=Sync to SYSCLKOUT  GPIO_Bit6_Qualification=Sync to SYSCLKOUT  GPIO_Bit7_Qualification=Sync to SYSCLKOUT  Qualification_Period=-1
  Gain : Gain  Gain=single(2.^(0:7))  ParamDataTypeStr=single
  Mux : Mux  Inputs=3
  Mux1 : Mux  Inputs=3
  Mux2 : Mux
  OR : Logic  Operator=OR  Inputs=1  AllPortsSameDT=off  OutDataTypeStr=boolean
  Sum of Elements : Sum  Inputs=+  OutDataTypeStr=uint8
  FLT : Outport
  FltCodeHw : Outport  Port=2
  wires:
  Digital Input/1 -> [SCP]
  Digital Input7/1 -> [OTP]
  Digital Input4/1 -> Data Type Conversion/1
  Digital Input5/1 -> Data Type Conversion1/1
  Digital Input6/1 -> Data Type Conversion2/1
  Mux1/1 -> [OVP]
  Data Type Conversion1/1 -> Mux1/2
  Data Type Conversion/1 -> Mux1/1
  Data Type Conversion2/1 -> Mux1/3
  Data Type Conversion5/1 -> Mux/3
  Data Type Conversion3/1 -> Mux/1
  Data Type Conversion4/1 -> Mux/2
  Digital Input3/1 -> Data Type Conversion5/1
  Digital Input2/1 -> Data Type Conversion4/1
  Digital Input1/1 -> Data Type Conversion3/1
  Mux/1 -> [OCP]
  Gain/1 -> Sum of Elements/1
  [OCP] -> Mux2/1
  [OVP] -> Mux2/2
  [SCP] -> Mux2/3
  [OTP] -> Mux2/4
  Mux2/1 -> OR/1, Gain/1
  OR/1 -> FLT/1  "Fail"
  Sum of Elements/1 -> FltCodeHw/1

== system GCI_Ctrl_PLL_C2000/C2000_SW/MnrErr/Monitoring ==
  ADC : Inport
  Irms : Inport  Port=2
  Vdc : Inport  Port=3
  Enable : EnablePort
  ADC_OORH : Subsystem  mask{Lim=Var.Diag_AdcOorHLim, LimN=single(-1), UorL=single(1), Tmon=Var.Diag_tOorHDtc}
      mask prompts: Lim "Upper Limit"; LimN "Lower Limit"; UorL "Selector Upper (1) or Lower (0)"; Tmon "Detection time (s)"
  ADC_OORL : Subsystem  mask{Lim=single(1), LimN=Var.Diag_AdcOorLLim, UorL=single(0), Tmon=Var.Diag_tOorLDtc}
      mask prompts: Lim "Upper Limit"; LimN "Lower Limit"; UorL "Selector Upper (1) or Lower (0)"; Tmon "Detection time (s)"
  Data Type Conversion : DataTypeConversion  OutDataTypeStr=single  SaturateOnIntegerOverflow=off  RndMeth=Floor
  Data Type Conversion1 : DataTypeConversion  OutDataTypeStr=uint16  SaturateOnIntegerOverflow=off  RndMeth=Floor
  Gain : Gain  Gain=single(2.^(0:13))  ParamDataTypeStr=single
  HvdcUOV : Subsystem  mask{Lim=Var.Diag_HvdcUOv, LimN=single(-1), UorL=single(1), Tmon=Var.Diag_tHvdcUOvDtc}
      mask prompts: Lim "Upper Limit"; LimN "Lower Limit"; UorL "Selector Upper (1) or Lower (0)"; Tmon "Detection time (s)"
  Mux : Mux
  OR : Logic  Operator=OR  Inputs=1  AllPortsSameDT=off  OutDataTypeStr=boolean
  RMS_OC : Subsystem  mask{Lim=Var.Diag_IrmsOc, LimN=single(-1), UorL=single(1), Tmon=Var.Diag_tIrmsDtc}
      mask prompts: Lim "Upper Limit"; LimN "Lower Limit"; UorL "Selector Upper (1) or Lower (0)"; Tmon "Detection time (s)"
  Sum of Elements : Sum  Inputs=+
  Failure : Outport  VectorParamsAs1DForOutWhenUnconnected=off
  FailCode : Outport  Port=2  VectorParamsAs1DForOutWhenUnconnected=off
  wires:
  ADC/1 -> Data Type Conversion/1  "ADC"
  ADC_OORH/1(err) -> Mux/1  "ORH"
  ADC_OORL/1(err) -> Mux/2  "ORL"
  OR/1 -> Failure/1  "Fail"
  Irms/1 -> RMS_OC/1(u)  "Irms"
  RMS_OC/1(err) -> Mux/3  "OC"
  HvdcUOV/1(err) -> Mux/4  "OV"
  Vdc/1 -> HvdcUOV/1(u)  "Vdc"
  Mux/1 -> Gain/1, OR/1  "MonErr"
  Data Type Conversion/1 -> ADC_OORL/1(u), ADC_OORH/1(u)  "DataTypeConversion"
  Gain/1 -> Sum of Elements/1
  Sum of Elements/1 -> Data Type Conversion1/1
  Data Type Conversion1/1 -> FailCode/1

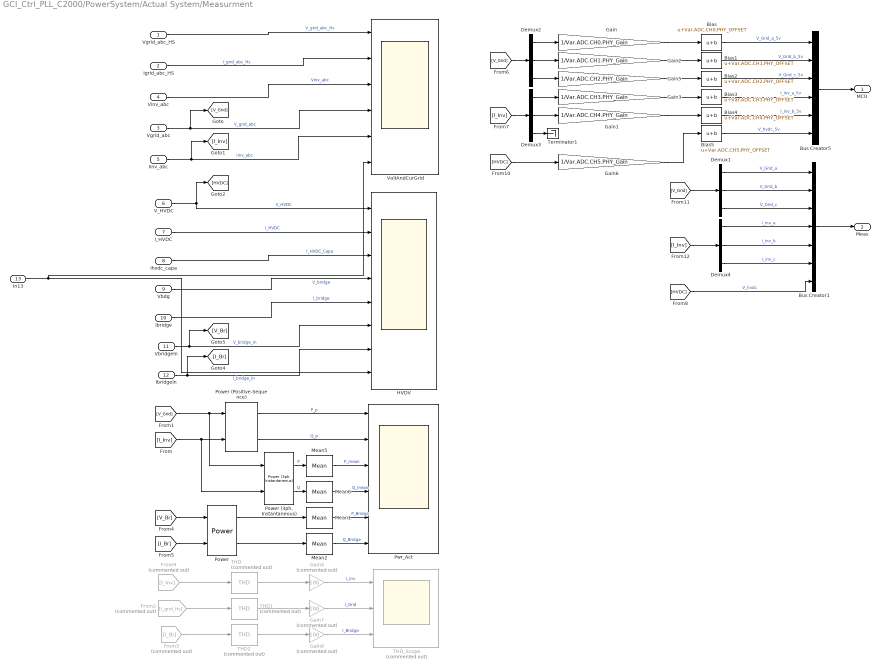
== system GCI_Ctrl_PLL_C2000/PowerSystem/Actual System/Measurment ==
  Vgrid_abc_HS : Inport
  Igrid_abc_HS : Inport  Port=2
  Vgrid_abc : Inport  Port=3
  Vinv_abc : Inport  Port=4
  Iinv_abc : Inport  Port=5
  V_HVDC : Inport  Port=6
  I_HVDC : Inport  Port=7
  Ihvdc_capa : Inport  Port=8
  Vbdg : Inport  Port=9
  Ibridge : Inport  Port=10
  VbridgeIn : Inport  Port=11
  IbridgeIn : Inport  Port=12
  In13 : Inport  Port=13
  Bias : Bias  Bias=Var.ADC.CH0.PHY_OFFSET  SaturateOnIntegerOverflow=off
  Bias1 : Bias  Bias=Var.ADC.CH1.PHY_OFFSET  SaturateOnIntegerOverflow=off
  Bias2 : Bias  Bias=Var.ADC.CH2.PHY_OFFSET  SaturateOnIntegerOverflow=off
  Bias3 : Bias  Bias=Var.ADC.CH3.PHY_OFFSET  SaturateOnIntegerOverflow=off
  Bias4 : Bias  Bias=Var.ADC.CH4.PHY_OFFSET  SaturateOnIntegerOverflow=off
  Bias5 : Bias  Bias=Var.ADC.CH5.PHY_OFFSET  SaturateOnIntegerOverflow=off
  Bus Creator1 : BusCreator  Inputs=7
  Bus Creator5 : BusCreator  Inputs=6
  Demux{1..4} (4 alike) : Demux  Outputs=3
  From2 : From  Commented=on  GotoTag=I_grid_Hs
  From3 : From  Commented=on  GotoTag=I_Br
  From9 : From  Commented=on  GotoTag=I_Inv
  Gain : Gain  Gain=1/Var.ADC.CH0.PHY_Gain
  Gain1 : Gain  Gain=1/Var.ADC.CH4.PHY_Gain
  Gain2 : Gain  Gain=1/Var.ADC.CH1.PHY_Gain
  Gain3 : Gain  Gain=1/Var.ADC.CH3.PHY_Gain
  Gain4 : Gain  Commented=on  Gain=100
  Gain5 : Gain  Gain=1/Var.ADC.CH2.PHY_Gain
  Gain6 : Gain  Gain=1/Var.ADC.CH5.PHY_Gain
  Gain7 : Gain  Commented=on  Gain=100
  Gain8 : Gain  Commented=on  Gain=100
  HVDV : Scope  NumInputPorts=8
  Mean{1..2,5..6} (4 alike) : spsMeanLib/Mean  Freq=double(Var.Grid.Frq )  Vinit=0  Ts=0
  Power : spsPowerLib/Power  Freq=60  Vinit=[1, 0]  Iinit=[1, 0]  Ts=0
  "Power (3ph, Instantaneous)" : spsPower3phInstantaneousLib/Power (3ph, Instantaneous)
  Power (Positive-Sequence) : spsPowerPositiveSequenceLib/Power (Positive-Sequence)  Freq=double(Var.Grid.Frq )  Vinit=[0, 0]  Iinit=[0, 0]  Ts=0
      settings: LibrarySourceBlock=|
      | sps_lib/Sensors and Measurements/Power
      | (Positive-Sequence)
  Pwr_Act : Scope  NumInputPorts=6
  THD : spsTHDLib/THD  Commented=on  Freq=double(Var.Grid.Frq )  Ts=0
  THD1 : spsTHDLib/THD  Commented=on  Freq=double(Var.Grid.Frq )  Ts=0
  THD2 : spsTHDLib/THD  Commented=on  Freq=double(Var.Grid.Frq )  Ts=0
  THD_Scope : Scope  Commented=on  NumInputPorts=3
  Terminator1 : Terminator
  VoltAndCurGrid : Scope  NumInputPorts=6
  MCU : Outport  VectorParamsAs1DForOutWhenUnconnected=off
  Meas : Outport  Port=2  VectorParamsAs1DForOutWhenUnconnected=off
  wires:
  Bias4/1 -> Bus Creator5/5  "I_inv_b_5v"
  Bias3/1 -> Bus Creator5/4  "I_inv_a_5v"
  Bias2/1 -> Bus Creator5/3  "V_Grid_c_5v"
  Gain5/1 -> Bias2/1
  Vgrid_abc/1 -> [V_Grid], VoltAndCurGrid/4  "V_grid_abc"
  From9/1 -> THD/1
  Mean6/1 -> Pwr_Act/4  "Q_mean"
  Mean5/1 -> Pwr_Act/3  "P_mean"
  "Power (3ph, Instantaneous)"/2 -> Mean6/1  "Q"
  "Power (3ph, Instantaneous)"/1 -> Mean5/1  "P"
  [V_Grid] -> "Power (3ph, Instantaneous)"/1, Power (Positive-Sequence)/1
  [I_Inv] -> "Power (3ph, Instantaneous)"/2, Power (Positive-Sequence)/2
  Gain4/1 -> THD_Scope/1  "I_inv"
  THD/1 -> Gain4/1
  Power (Positive-Sequence)/2 -> Pwr_Act/2  "Q_p"
  Power (Positive-Sequence)/1 -> Pwr_Act/1  "P_p"
  Demux3/1 -> Gain3/1
  Demux3/3 -> Terminator1/1
  Gain2/1 -> Bias1/1
  Demux2/3 -> Gain5/1
  Demux2/2 -> Gain2/1
  Gain/1 -> Bias/1
  Ibridge/1 -> HVDV/5  "I_bridge"
  Vbdg/1 -> HVDV/4  "V_bridge"
  Ihvdc_capa/1 -> HVDV/3  "I_HVDC_Capa"
  Bus Creator5/1 -> MCU/1
  Bias/1 -> Bus Creator5/1  "V_Grid_a_5v"
  Bias1/1 -> Bus Creator5/2  "V_Grid_b_5v"
  Gain3/1 -> Bias3/1
  Gain1/1 -> Bias4/1
  Demux3/2 -> Gain1/1
  Demux2/1 -> Gain/1
  [I_Inv] -> Demux3/1
  [V_Grid] -> Demux2/1
  I_HVDC/1 -> HVDV/2  "I_HVDC"
  V_HVDC/1 -> [HVDC], HVDV/1  "V_HVDC"
  Vinv_abc/1 -> VoltAndCurGrid/3  "Vinv_abc"
  Iinv_abc/1 -> VoltAndCurGrid/5, [I_Inv]  "Iinv_abc"
  [HVDC] -> Gain6/1
  Gain6/1 -> Bias5/1
  Bias5/1 -> Bus Creator5/6  "V_hvdc_5v"
  Vgrid_abc_HS/1 -> VoltAndCurGrid/1  "V_grid_abc_Hs"
  Igrid_abc_HS/1 -> VoltAndCurGrid/2  "I_grid_abc_Hs"
  From2/1 -> THD1/1
  THD1/1 -> Gain7/1
  Gain7/1 -> THD_Scope/2  "I_Grid"
  VbridgeIn/1 -> [V_Br], HVDV/6  "V_bridge_In"
  IbridgeIn/1 -> [I_Br], HVDV/7  "I_bridge_In"
  THD2/1 -> Gain8/1
  From3/1 -> THD2/1
  Gain8/1 -> THD_Scope/3  "I_Bridge"
  Power/1 -> Mean1/1
  Power/2 -> Mean2/1
  [I_Br] -> Power/2
  [V_Br] -> Power/1
  Mean1/1 -> Pwr_Act/5  "P_Bridge"
  Mean2/1 -> Pwr_Act/6  "Q_Bridge"
  In13/1 -> VoltAndCurGrid/6, HVDV/8
  [HVDC] -> Bus Creator1/7  "V_hvdc"
  [V_Grid] -> Demux1/1
  [I_Inv] -> Demux4/1
  Demux1/1 -> Bus Creator1/1  "V_Grid_a"
  Demux4/2 -> Bus Creator1/5  "I_inv_b"
  Demux1/2 -> Bus Creator1/2  "V_Grid_b"
  Demux1/3 -> Bus Creator1/3  "V_Grid_c"
  Demux4/3 -> Bus Creator1/6  "I_inv_c"
  Demux4/1 -> Bus Creator1/4  "I_inv_a"
  Bus Creator1/1 -> Meas/1

== system GCI_Ctrl_PLL_C2000/PowerSystem/Actual System/PWMGen2 ==
  Duty : Inport
  Compare To Constant : simulink/Logic and Bit Operations/Compare To Constant  relop=>  const=99.9  OutDataTypeStr=boolean
  Constant : Constant  Value=0.5
  Deadtime : Subsystem  Commented=on
  Gain1 : Gain  Gain=2
  GreaterThan : RelationalOperator  Operator=>  RndMeth=Simplest  InputSameDT=off
  GreaterThan1 : RelationalOperator  Operator=>  RndMeth=Simplest  InputSameDT=off
  Mux : Mux  Inputs=2
  Repeating Sequence : simulink/Sources/Repeating Sequence  rep_seq_t=[0 0.5/Var.PWM.Freq 1/Var.PWM.Freq]  rep_seq_y=[0 100 0]
  Scope : Scope  NumInputPorts=5
  Selector : Selector  InputPortWidth=6  IndexOptions=Index vector (dialog)  Indices=[1 4 2 5 3 6]  OutputSizes=1
  Selector1 : Selector  InputPortWidth=6  IndexOptions=Index vector (dialog)  Indices=[1 2 3]  OutputSizes=1
  Selector2 : Selector  InputPortWidth=6  IndexOptions=Index vector (dialog)  Indices=[4 5 6]  OutputSizes=1
  Subtract : Sum  Inputs=+-
  PWM : Outport  VectorParamsAs1DForOutWhenUnconnected=off
  MeasTrig : Outport  Port=2  VectorParamsAs1DForOutWhenUnconnected=off
  wires:
  Selector/1 -> Subtract/1
  GreaterThan1/1 -> Mux/2
  GreaterThan/1 -> Mux/1
  Selector2/1 -> GreaterThan1/2
  Selector1/1 -> GreaterThan/1, Scope/2
  Duty/1 -> Selector1/1, Selector2/1, Scope/1
  Subtract/1 -> Gain1/1
  Constant/1 -> Subtract/2
  Repeating Sequence/1 -> GreaterThan/2, Scope/3, Compare To Constant/1, GreaterThan1/1
  Gain1/1 -> PWM/1, Scope/4
  Mux/1 -> Selector/1
  Compare To Constant/1 -> MeasTrig/1, Scope/5

== system GCI_Ctrl_PLL_C2000/PowerSystem/Actual System/Triggered Subsystem ==
  In1 : Inport
  Trigger : TriggerPort  VariantControl=Variant
  Out1 : Outport  VectorParamsAs1DForOutWhenUnconnected=off
  wires:
  In1/1 -> Out1/1

== system GCI_Ctrl_PLL_C2000/PowerSystem/Meas/Fault Injection ==
  3PhaseToGnd : Subsystem  VariantControl="Var.Sim.FltInj == \"Three Phase Gnd\""  mask{Frq=double(Var.Grid.Frq ), FrqStp=[-4 6.5], FrqStpT=[1 1], Mag=1, MagStpPerc=[0.1 0.1 0.1], MagStpT=0.4, Pha=[0 -120 120], PhaStpPerc=20, PhaStpT=3, HarmOrd=[5 7], Harm=[-5 2.5]./100, HarmStp=1, IntHarmOrd=[5.4 7.3], IntHarm=[8 4]./100, IntHarmStp=1, DcOff=[ 0 0 0]./100}
      mask prompts: Frq "Frequency"; FrqStp "Frequency Step Hz"; FrqStpT "Frequency Step Time"; Mag "Magnitude"; MagStpPerc "Magnitude Step %"; MagStpT "Magnitude Step Time"; Pha "Phase"; PhaStpPerc "Phase Step Deg"; PhaStpT "Phase Step Time"; HarmOrd "Harmonic Order ex(3rd, 5th,...)"; Harm "Harmonics Percentage"; HarmStp "Harmonics Step Time"; IntHarmOrd "Inter Harmonic Order ex(5.4th, 7.3th,...)"; IntHarm "Inter Harmonics Percentage"; IntHarmStp "Inter Harmonics Step Time"; DcOff "DC Offcet Percent"
      mask DialogControl Container3 Prompt: Freq Step Parameters
      mask DialogControl Container4 Prompt: Mag Step Parameters
      mask DialogControl Container5 Prompt: Phase Step Parameters
      mask DialogControl Container6 Prompt: Harmonics
      mask DialogControl Container7 Prompt: Inter Harmonics
      mask DialogControl Container8 Prompt: DC OffSet
  FreqVar : Subsystem  VariantControl=Var.Sim.FltInj == 3  mask{Frq=double(Var.Grid.Frq ), FrqStp=[-4 6.5], FrqStpT=[0.5 0.7], Mag=1, MagStpPerc=[0.2 0.2 1], MagStpT=1, Pha=[0 -120 120], PhaStpPerc=20, PhaStpT=3, HarmOrd=[5 7], Harm=[6.5 5.5]./100, HarmStp=3, IntHarmOrd=[3.4 5.6], IntHarm=[3.5 -4]./100, IntHarmStp=3, DcOff=[ 6 4 5.2]./100}
      mask prompts: Frq "Frequency"; FrqStp "Frequency Step Hz"; FrqStpT "Frequency Step Time"; Mag "Magnitude"; MagStpPerc "Magnitude Step %"; MagStpT "Magnitude Step Time"; Pha "Phase"; PhaStpPerc "Phase Step Deg"; PhaStpT "Phase Step Time"; HarmOrd "Harmonic Order ex(3rd, 5th,...)"; Harm "Harmonics Percentage"; HarmStp "Harmonics Step Time"; IntHarmOrd "Inter Harmonic Order ex(5.4th, 7.3th,...)"; IntHarm "Inter Harmonics Percentage"; IntHarmStp "Inter Harmonics Step Time"; DcOff "DC Offcet Percent"
      mask DialogControl Container3 Prompt: Freq Step Parameters
      mask DialogControl Container4 Prompt: Mag Step Parameters
      mask DialogControl Container5 Prompt: Phase Step Parameters
      mask DialogControl Container6 Prompt: Harmonics
      mask DialogControl Container7 Prompt: Inter Harmonics
      mask DialogControl Container8 Prompt: DC OffSet
  Harm : Subsystem  VariantControl="Var.Sim.FltInj == \"Harmonics Injection\""  mask{Frq=double(Var.Grid.Frq ), FrqStp=[-4 6.5], FrqStpT=[1 1], Mag=1, MagStpPerc=[0.2 1 0.2], MagStpT=0.7, Pha=[0 -120 120], PhaStpPerc=20, PhaStpT=3, HarmOrd=[5 7], Harm=[-5 2.5]./100, HarmStp=0.6, IntHarmOrd=[5.4 7.3], IntHarm=[8 4]./100, IntHarmStp=0.65, DcOff=[ 0 0 0]./100}
      mask prompts: Frq "Frequency"; FrqStp "Frequency Step Hz"; FrqStpT "Frequency Step Time"; Mag "Magnitude"; MagStpPerc "Magnitude Step %"; MagStpT "Magnitude Step Time"; Pha "Phase"; PhaStpPerc "Phase Step Deg"; PhaStpT "Phase Step Time"; HarmOrd "Harmonic Order ex(3rd, 5th,...)"; Harm "Harmonics Percentage"; HarmStp "Harmonics Step Time"; IntHarmOrd "Inter Harmonic Order ex(5.4th, 7.3th,...)"; IntHarm "Inter Harmonics Percentage"; IntHarmStp "Inter Harmonics Step Time"; DcOff "DC Offcet Percent"
      mask DialogControl Container3 Prompt: Freq Step Parameters
      mask DialogControl Container4 Prompt: Mag Step Parameters
      mask DialogControl Container5 Prompt: Phase Step Parameters
      mask DialogControl Container6 Prompt: Harmonics
      mask DialogControl Container7 Prompt: Inter Harmonics
      mask DialogControl Container8 Prompt: DC OffSet
  TwoPhaseFault : Subsystem  VariantControl="Var.Sim.FltInj == \"Two Phase Flt\""  mask{Frq=double(Var.Grid.Frq ), FrqStp=[-4 6.5], FrqStpT=[1 1], Mag=1, MagStpPerc=[2/3 1/6 2/3], MagStpT=0.75, Pha=[0 -120 120], PhaStpPerc=20, PhaStpT=3, HarmOrd=[5 7], Harm=[-5 2.5]./100, HarmStp=1, IntHarmOrd=[5.4 7.3], IntHarm=[8 4]./100, IntHarmStp=1, DcOff=[ 0 0 0]./100, DcStpT=0}
      mask prompts: Frq "Frequency"; FrqStp "Frequency Step Hz"; FrqStpT "Frequency Step Time"; Mag "Magnitude"; MagStpPerc "Magnitude Step %"; MagStpT "Magnitude Step Time"; Pha "Phase"; PhaStpPerc "Phase Step Deg"; PhaStpT "Phase Step Time"; HarmOrd "Harmonic Order ex(3rd, 5th,...)"; Harm "Harmonics Percentage"; HarmStp "Harmonics Step Time"; IntHarmOrd "Inter Harmonic Order ex(5.4th, 7.3th,...)"; IntHarm "Inter Harmonics Percentage"; IntHarmStp "Inter Harmonics Step Time"; DcOff "DC Offset Percent"; DcStpT "DC Offset Step Time"
      mask DialogControl Container3 Prompt: Freq Step Parameters
      mask DialogControl Container4 Prompt: Mag Step Parameters
      mask DialogControl Container5 Prompt: Phase Step Parameters
      mask DialogControl Container6 Prompt: Harmonics
      mask DialogControl Container7 Prompt: Inter Harmonics
      mask DialogControl Container8 Prompt: DC OffSet
  Wave : Outport  VectorParamsAs1DForOutWhenUnconnected=off
